simulink model "MAS_Full_State_AS_1"  (R2021b)
settings: Solver=VariableStepAuto  StartTime=0.0  StopTime=1000  RelTol=1e-3
model workspace (MAT data in the model file):
  A = [0  1  0; -1  0  1; 0  -1  0]
  B = [0  0; 1  0; 1  -1]
  C = [0  1  2; 0  0  -1; 1  0  1]
  D = [0  0; 0  0; 0  0]
libraries: cstblocks x6
settings Model: Creator=lenovo  LastModifiedBy=lenovo

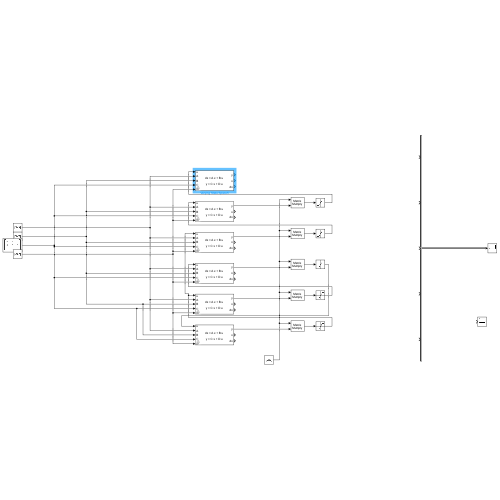
[thumbnail: Simulink's stored preview of the top-level diagram]
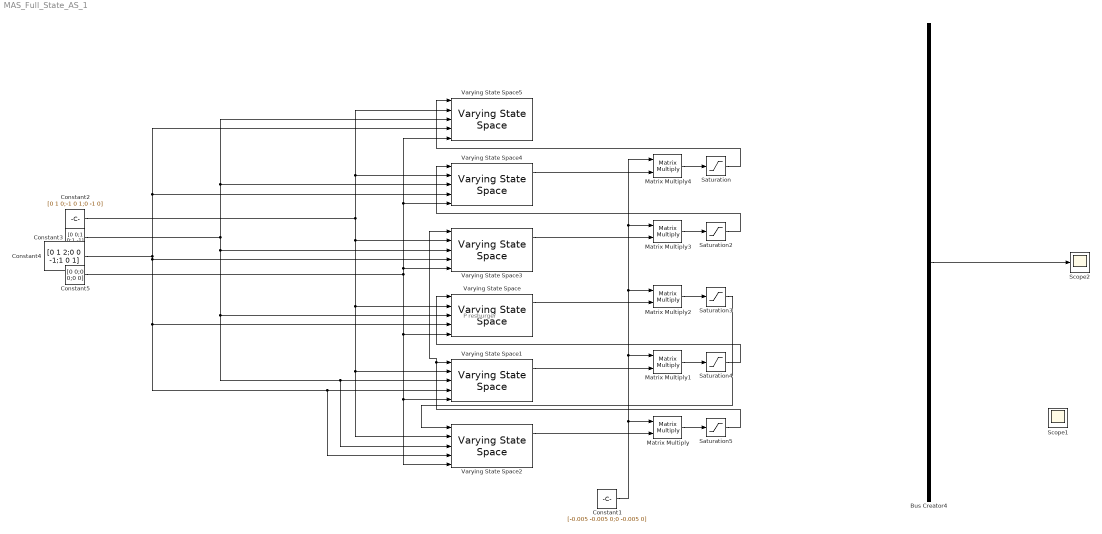
== system MAS_Full_State_AS_1 ==
  note: P resburger
  Bus Creator4 : BusCreator  Inputs=5
  Constant1 : Constant  Value=[-0.005 -0.005 0;0 -0.005 0]  VectorParams1D=off
  Constant2 : Constant  Value=[0 1 0;-1 0 1;0 -1 0]
  Constant3 : Constant  Value=[0 0;1 0;1 -1]
  Constant4 : Constant  Value=[0 1 2;0 0 -1;1 0 1]  VectorParams1D=off
  Constant5 : Constant  Value=[0 0;0 0;0 0]  VectorParams1D=off
  Matrix Multiply{,1..4} (5 alike) : Product  Multiplication=Matrix(*)
  Saturation{,2..5} (5 alike) : Saturate  UpperLimit=0.1  LowerLimit=-0.1
  Scope1 : Scope
  Scope2 : Scope
  Varying State Space : cstblocks/Linear Parameter Varying/Varying State Space  x0=[-2;1;1]  xNames=''  OutputX=on  OutputDX=on
  Varying State Space1 : cstblocks/Linear Parameter Varying/Varying State Space  x0=[2;2;-1]  xNames=''  OutputX=on  OutputDX=on
  Varying State Space2 : cstblocks/Linear Parameter Varying/Varying State Space  x0=[-1;1;2]  xNames=''  OutputX=on  OutputDX=on
  Varying State Space3 : cstblocks/Linear Parameter Varying/Varying State Space  x0=[-1;-1;-2]  xNames=''  OutputX=on  OutputDX=on
  Varying State Space4 : cstblocks/Linear Parameter Varying/Varying State Space  x0=[-3;2;-1]  xNames=''  OutputX=on  OutputDX=on
  Varying State Space5 : cstblocks/Linear Parameter Varying/Varying State Space  x0=[3;-2;-1]  xNames=''  OutputX=on  OutputDX=on
  wires:
  Bus Creator4/1 -> Scope2/1
  Constant2/1 -> Varying State Space2/2, Varying State Space1/2, Varying State Space/2, Varying State Space3/2, Varying State Space4/2, Varying State Space5/2
  Constant3/1 -> Varying State Space3/3, Varying State Space2/3, Varying State Space1/3, Varying State Space/3, Varying State Space4/3, Varying State Space5/3
  Constant4/1 -> Varying State Space/4, Varying State Space2/4, Varying State Space1/4, Varying State Space3/4, Varying State Space4/4, Varying State Space5/4
  Constant5/1 -> Varying State Space/5, Varying State Space2/5, Varying State Space1/5, Varying State Space5/5, Varying State Space4/5, Varying State Space3/5
  Constant1/1 -> Matrix Multiply4/1, Matrix Multiply3/1, Matrix Multiply2/1, Matrix Multiply1/1, Matrix Multiply/1
  Varying State Space2/1 -> Matrix Multiply/2
  Varying State Space1/1 -> Matrix Multiply1/2
  Varying State Space/1 -> Matrix Multiply2/2
  Varying State Space3/1 -> Matrix Multiply3/2
  Varying State Space4/1 -> Matrix Multiply4/2
  Matrix Multiply/1 -> Saturation5/1
  Matrix Multiply1/1 -> Saturation4/1
  Matrix Multiply2/1 -> Saturation3/1
  Matrix Multiply3/1 -> Saturation2/1
  Matrix Multiply4/1 -> Saturation/1
  Saturation5/1 -> Varying State Space3/1, Varying State Space1/1
  Saturation4/1 -> Varying State Space/1
  Saturation3/1 -> Varying State Space2/1
  Saturation2/1 -> Varying State Space4/1
  Saturation/1 -> Varying State Space5/1
